simulink model "rx"  (R2013a)
settings: Solver=ode45  StartTime=0.0  StopTime=10.0  RelTol=1e-3
undefined symbols (not defined in the file or in its folder): gcbh, xlBlockLoadCallback, xlGetNormalizedPeriod
libraries: xbsIndex_r4 x68, xbsEDKLib_r4 x1
(part 1 of 2)
settings Model: Creator=apple  LastModifiedBy=rcagley
settings OptimizationCC: ExpressionDepthLimit=2147483647

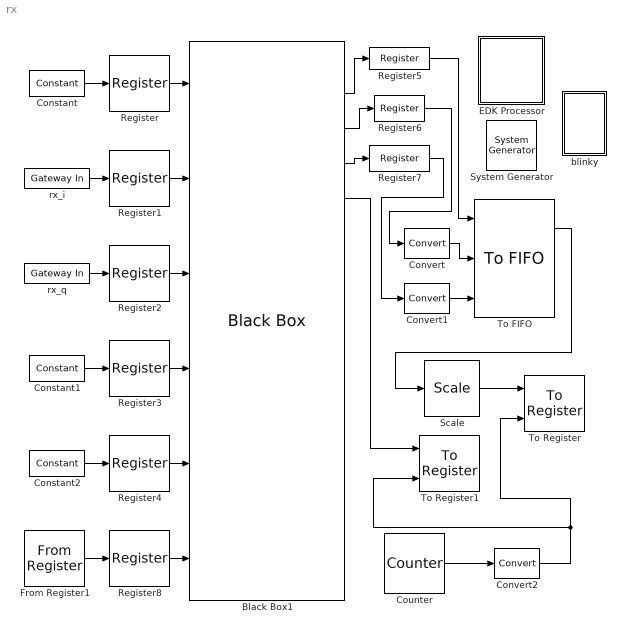
== system rx ==
  " System Generator" : xbsIndex_r4/ System Generator  Tag=genX  xilinxfamily=zynq  part=xc7z020  speed=-1  package=clg484  synthesis_tool=XST  clock_wrapper=Clock Enables  directory=./netlist  proj_type=Project Navigator  Synth_file=XST Defaults  Impl_file=ISE Defaults  testbench=off  simulink_period=1  sysclk_period=50  dcm_input_clock_period=10  incr_netlist=off  trim_vbits=Everywhere in SubSystem  dbl_ovrd=According to Block Masks  core_generation=According to Block Masks  run_coregen=off  deprecated_control=off  eval_field=0  block_type=sysgen
  Black Box1 : xbsIndex_r4/Black Box  init_code=qpsk_rx_FixPt_xsgbbxcfg  sim_method=Inactive  verbose=off  block_type=blackbox2
  Constant : xbsIndex_r4/Constant  const=0  gui_display_data_type=Fixed-point  arith_type=Unsigned  n_bits=1  bin_pt=0  preci_type=Single  exp_width=8  frac_width=24  explicit_period=on  period=1  equ=P=C  opselect=C  inp2=PCIN>>17  opr=+  inp1=P  carry=CIN  dbl_ovrd=off  block_type=constant
  Constant1 : xbsIndex_r4/Constant  const=floor(.01*2^12)  gui_display_data_type=Fixed-point  arith_type=Unsigned  n_bits=12  bin_pt=0  preci_type=Single  exp_width=8  frac_width=24  explicit_period=on  period=1  equ=P=C  opselect=C  inp2=PCIN>>17  opr=+  inp1=P  carry=CIN  dbl_ovrd=off  block_type=constant
  Constant2 : xbsIndex_r4/Constant  const=floor(.01*8*2^12)  gui_display_data_type=Fixed-point  arith_type=Unsigned  n_bits=12  bin_pt=0  preci_type=Single  exp_width=8  frac_width=24  explicit_period=on  period=1  equ=P=C  opselect=C  inp2=PCIN>>17  opr=+  inp1=P  carry=CIN  dbl_ovrd=off  block_type=constant
  Convert : xbsIndex_r4/Convert  gui_display_data_type=Boolean  arith_type=Boolean  n_bits=16  bin_pt=14  float_type=Single  exp_bits=8  fraction_bits=24  quantization=Truncate  overflow=Wrap  en=off  latency=0  dbl_ovrd=off  pipeline=off  block_type=convert
  Convert1 : xbsIndex_r4/Convert  gui_display_data_type=Boolean  arith_type=Boolean  n_bits=16  bin_pt=14  float_type=Single  exp_bits=8  fraction_bits=24  quantization=Truncate  overflow=Wrap  en=off  latency=0  dbl_ovrd=off  pipeline=off  block_type=convert
  Convert2 : xbsIndex_r4/Convert  gui_display_data_type=Boolean  arith_type=Boolean  n_bits=16  bin_pt=14  float_type=Single  exp_bits=8  fraction_bits=24  quantization=Truncate  overflow=Wrap  en=off  latency=0  dbl_ovrd=off  pipeline=off  block_type=convert
  Counter : xbsIndex_r4/Counter  cnt_type=Free Running  cnt_to=Inf  operation=Up  start_count=0  cnt_by_val=1  arith_type=Unsigned  n_bits=1  bin_pt=0  load_pin=off  rst=off  en=off  explicit_period=on  period=1  dbl_ovrd=off  use_behavioral_HDL=off  implementation=Fabric  block_type=counter
  EDK Processor : Subsystem  LoadFcn=xlBlockLoadCallback(gcbh);  mask(Xilinx EDK Processor Block){mode=EDK pcore generation, xmp=, MemVisToProc=<qt bgcolor="#FFFFFF"><div><img src="C:/Xilinx/14.4/ISE_DS/ISE/sysgen/data/images/registerplus.gif"> &lt;&lt;percent_full&gt;&gt;<br></div><div><img src="C:/Xilinx/14.4/ISE_DS/ISE/sysgen/data/images/registerplus.gif"> &lt;&lt;mcu_rx_ready&gt;&gt;<br></div><div><img src="C:/Xilinx/14.4/ISE_DS/ISE/sysgen/data/images/registerplus.gif"> &lt;&lt;num_bytes_ready&gt;&gt;<br></div><div><img src="C:/Xilinx/14.4/ISE_DS/ISE/sysgen/data/images/fifoplus.gif"> &lt;&lt;rx_fifo&gt;&gt;<br></div></qt>, AvailableMemories=<empty>, portInterfaceTable={'exposed'=>[],'portdir'=>[],'portname'=>[],'shortname'=>[]}, bus_type_sgadvanced=, bus_type=AXI, baseaddr=0x80000000, baseaddr_lock_sgadvanced=, baseaddr_lock=off, dual_clock_sgadvanced=, dual_clock=on, reg_readback_sgadvanced=, reg_readback=off, ucf_file=, inheritDeviceType_sgadvanced=, inheritDeviceType=off, elf_file=, codebug_sgadvanced=, codebug=on, clock_name=plb, internalPortList={}, resetPolarity=0, memxtable={'mladdr'=>[0.00000000000000000,0.00000000000000000,1.00000000000000000,-1.00000000000000000],'mlist'=>['rx/To Register','rx/From Register1','rx/To Register1','rx/To FIFO'],'mlname'=>['\'percent_full\'','\'mcu_rx_ready\'','\'num_bytes_ready\'','\'rx_fifo\''],'mlstate'=>[0.00000000000000000,0.00000000000000000,0.00000000000000000,0.00000000000000000]}, procinfo={}, memmapdirty=off, blockname=, xpsintstyle=default, has_advanced_control=0, sggui_pos=-1,-1,-1,-1, block_type=edkprocessor, block_version=2.7, sg_icon_stat=62,64,0,0,white,blue,0,58c5b5770fe5f7c311f53dbc6e73f0f6,right,,[ ],[ ], sg_mask_display=|, sg_list_contents={'table'=>{'AvailableMemories'=>'popup(<empty>)'}}, sg_blockgui_xml=}
      mask sg_mask_display=|
      | fprintf('','COMMENT: begin icon graphics');
      | patch([0 62 62 0 0 ],[0 0 64 64 0 ],[0.77 0.82 0.91 ]);
      | plot([0 62 62 0 0 ],[0 0 64 64 0 ]);
      | patch([13.2 24.76 32.76 40.76 48.76 32.76 21.2 13.2 ],[40.88 40.88 48.88 40.88 48.88 48.88 48.88 40.88 ],[1 1 1 ]);
      | patch([21.2 32.76 24.76 13.2 21.2 ],[32.88 32.88 40.88 40.88 32.88 ],[0.931 0.946 0.973 ]);
      | patch([13.2 24.76 32.76 21.2 13.2 ],[24.88 24.88 32.88 32.88 24.88 ],[1 1 1 ]);
      | patch([21.2 48.76 40.76 32.76 24.76 13.2 21.2 ],[16.88 16.88 24.88 16.88 24.88 24.88 16.88 ],[0.931 0.946 0.973 ]);
      | fprintf('','COMMENT: end icon graphics');
      | fprintf('','COMMENT: begin icon text');
      |
      | fprintf('','COMMENT: end icon text');
      mask prompts: mode "Configure Processor for"; xmp "XPS Project"; MemVisToProc ""; AvailableMemories "Available Memories"; portInterfaceTable ""; bus_type_sgadvanced ""; bus_type "Bus Type"; baseaddr "Base Address"; baseaddr_lock_sgadvanced ""; baseaddr_lock "Lock"; dual_clock_sgadvanced ""; dual_clock "Dual Clocks"; reg_readback_sgadvanced ""; reg_readback "Register Read-Back"; ucf_file "Constraint File"; inheritDeviceType_sgadvanced ""; inheritDeviceType "Inherit Device Type"; elf_file "Initial Program"; codebug_sgadvanced ""; codebug "Enable Co-Debug with Xilinx SDK (Beta)"; clock_name ""; internalPortList ""; resetPolarity ""; memxtable ""; procinfo ""; memmapdirty ""; blockname ""; xpsintstyle ""; has_advanced_control ""; sggui_pos ""; block_type ""; block_version ""; sg_icon_stat ""; sg_mask_display ""; sg_list_contents ""; sg_blockgui_xml ""
      mask help: Xilinx EDK Processor
      mask init:
      | try
      |   tmp_gcb = gcb;
      |   tmp_gcbh = gcbh;
      |   if (strcmp('SysGenIndex',get_param(bdroot(tmp_gcbh),'tag')) && ~isempty(regexp(bdroot(tmp_gcb), '^xbs', 'once')))
      |     return;
      |   end;
      |   xlMungeMaskParams;
      | 
      |   block_type='edkprocessor';
      | 
      |   serialized_declarations = '{''block_type''=>''String''}';
      |   xledkprocessor_init();
      |   ptable_ = xlblockprep(get_param(tmp_gcb, 'MaskWSVariables'));
      |   try
      |     xlBlockMoveCallback(tmp_gcbh);
      |   catch 
      |      clear global xl_updateicon_recursion_guard;
      |   end;
      | catch
      |   global dbgsysgen;
      |   if(~isempty(dbgsysgen) && dbgsysgen)
      |     e = regexprep(lasterr, '\n', '\nError: ');
      |     disp(['Error: While running MaskInit code on block ' tmp_gcb ': ' e]);
      |     error(e);
      |   end
      | end
      settings: CopyFcn=xlProcBlockCopyCallback(gcbh);xlBlockMoveCallback(gcbh);  DeleteFcn=xlDestroyGui(gcbh);  ModelCloseFcn=xlDestroyGui(gcbh);  PreSaveFcn=xlBlockPreSaveCallback(gcbh);  PostSaveFcn=xlBlockPostSaveCallback(gcbh);  DestroyFcn=xlDestroyGui(gcbh);  OpenFcn=bh=gcbh;xlProcBlockCallbacks('populatesharedmemorylistbox',bh);xlOpenGui(bh, 'edkprocessor_gui.xml', @xlProcBlockEnablement, @xlProcBlockAction);  CloseFcn=xlDestroyGui(gcbh);  MoveFcn=xlBlockMoveCallback(gcbh);
      mask Help: eval('');xlDoc('-book','sysgen','-topic','EDK_Processor');
      mask TypeOptions mode: EDK pcore generation | HDL netlisting
      mask TypeOptions bus_type: AXI | PLB
      mask Display:
      | fprintf('','COMMENT: begin icon graphics');
      | patch([0 62 62 0 0 ],[0 0 64 64 0 ],[0.77 0.82 0.91 ]);
      | plot([0 62 62 0 0 ],[0 0 64 64 0 ]);
      | patch([13.2 24.76 32.76 40.76 48.76 32.76 21.2 13.2 ],[40.88 40.88 48.88 40.88 48.88 48.88 48.88 40.88 ],[1 1 1 ]);
      | patch([21.2 32.76 24.76 13.2 21.2 ],[32.88 32.88 40.88 40.88 32.88 ],[0.931 0.946 0.973 ]);
      | patch([13.2 24.76 32.76 21.2 13.2 ],[24.88 24.88 32.88 32.88 24.88 ],[1 1 1 ]);
      | patch([21.2 48.76 40.76 32.76 24.76 13.2 21.2 ],[16.88 16.88 24.88 16.88 24.88 24.88 16.88 ],[0.931 0.946 0.973 ]);
      | fprintf('','COMMENT: end icon graphics');
      | fprintf('','COMMENT: begin icon text');
      | disp('');
      | 
      | fprintf('','COMMENT: end icon text');
  From Register1 : xbsIndex_r4/From Register  shared_memory_name='mcu_rx_ready'  init=0  period=1  ownership=Owned and initialized elsewhere  gui_display_data_type=Fixed-point  arith_type=Unsigned  n_bits=1  bin_pt=0  preci_type=Single  dbl_ovrd=off  block_type=fromreg
      settings: AttributesFormatString=<< %<shared_memory_name> >>  infoedit="Register block that reads data to a shared memory register.  Delay of one sample period."
  Register{,1..8} (9 alike) : xbsIndex_r4/Register  init=0  rst=off  en=off  dbl_ovrd=off  block_type=register
  Scale : xbsIndex_r4/Scale  scale_factor=10  dbl_ovrd=off  block_type=scale
  To FIFO : xbsIndex_r4/To FIFO  shared_memory_name='rx_fifo'  ownership=Locally owned  mem_type=Block RAM  performance_options=Standard_FIFO  infoedit1=Available only for V4, V5, V6, V7, K7, A7 and Zynq devices.  embedded_registers=off  depth=1K  percent_nbits=10  has_arst=on  use_percent_full_port=on  explicit_data_type=on  gui_display_data_type=Fixed-point  arith_type=Unsigned  n_bits=8  bin_pt=0  preci_type=Single  dbl_ovrd=off  block_type=tofifo
      settings: AttributesFormatString=<< %<shared_memory_name> >>  infoedit=First-in-first-out (FIFO) block that writes FIFO data to shared memory storage.
  To Register : xbsIndex_r4/To Register  shared_memory_name='percent_full'  init=0  ownership=Locally owned and initialized  explicit_data_type=on  gui_display_data_type=Fixed-point  arith_type=Unsigned  n_bits=10  bin_pt=0  preci_type=Single  dbl_ovrd=off  block_type=toreg
      settings: AttributesFormatString=<< %<shared_memory_name> >>  infoedit="Register block that writes data to a shared memory register.  Delay of one sample period."
  To Register1 : xbsIndex_r4/To Register  shared_memory_name='num_bytes_ready'  init=0  ownership=Locally owned and initialized  explicit_data_type=on  gui_display_data_type=Fixed-point  arith_type=Unsigned  n_bits=9  bin_pt=0  preci_type=Single  dbl_ovrd=off  block_type=toreg
      settings: AttributesFormatString=<< %<shared_memory_name> >>  infoedit="Register block that writes data to a shared memory register.  Delay of one sample period."
  blinky : Subsystem
  rx_i : xbsIndex_r4/Gateway In  gui_display_data_type=Fixed-point  arith_type="Signed  (2's comp)"  n_bits=12  bin_pt=0  preci_type=Single  exp_width=8  frac_width=24  quantization="Round  (unbiased: +/- Inf)"  overflow=Saturate  period=1  dbl_ovrd=off  timing_constraint=None  locs_specified=off  LOCs={}  UseAsADC=off  ADCChannel='1'  inherit_from_input=off  hdl_port=on  block_type=gatewayin
  rx_q : xbsIndex_r4/Gateway In  gui_display_data_type=Fixed-point  arith_type="Signed  (2's comp)"  n_bits=12  bin_pt=0  preci_type=Single  exp_width=8  frac_width=24  quantization="Round  (unbiased: +/- Inf)"  overflow=Saturate  period=1  dbl_ovrd=off  timing_constraint=None  locs_specified=off  LOCs={}  UseAsADC=off  ADCChannel='1'  inherit_from_input=off  hdl_port=on  block_type=gatewayin
  wires:
  rx_q/1 -> Register2/1
  rx_i/1 -> Register1/1
  Black Box1/3 -> Register6/1
  Black Box1/4 -> Register7/1
  Convert/1 -> To FIFO/2
  Register/1 -> Black Box1/1
  Register2/1 -> Black Box1/3
  Register3/1 -> Black Box1/4
  Register4/1 -> Black Box1/5
  Register5/1 -> To FIFO/1
  Register6/1 -> Convert/1
  Register1/1 -> Black Box1/2
  Constant/1 -> Register/1
  Constant1/1 -> Register3/1
  Constant2/1 -> Register4/1
  Black Box1/2 -> Register5/1
  Register7/1 -> Convert1/1
  Convert1/1 -> To FIFO/3
  To FIFO/1 -> Scale/1
  Register8/1 -> Black Box1/6
  From Register1/1 -> Register8/1
  Counter/1 -> Convert2/1
  Convert2/1 -> To Register/2, To Register1/2
  Scale/1 -> To Register/1
  Black Box1/5 -> To Register1/1
